simulink model "PWM_single_fixed"  (R2023a)
settings: Solver=VariableStepAuto  StartTime=0.0  StopTime=5  RelTol=1e-3
libraries: simulink x4
settings Model: Creator=Dell  LastModifiedBy=dhana
settings RTWCC: GPUComputeCapability=5.0

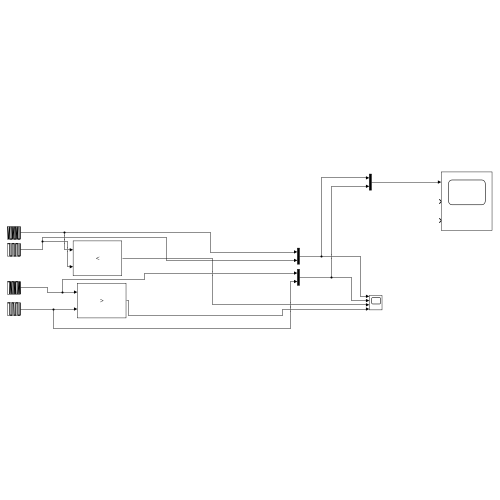
[thumbnail: Simulink's stored preview of the top-level diagram]
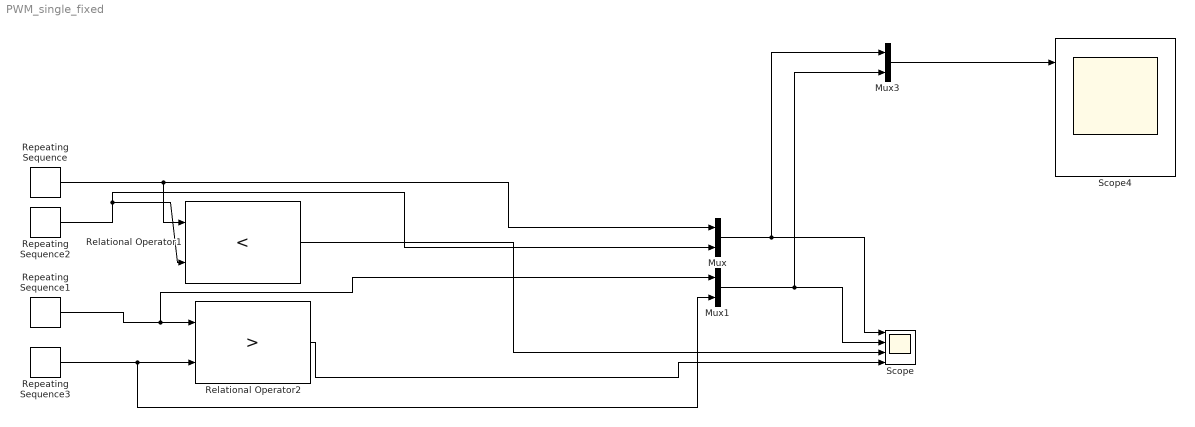
== system PWM_single_fixed ==
  Mux : Mux  Inputs=2
  Mux1 : Mux  Inputs=2
  Mux3 : Mux  Inputs=2
  Relational Operator1 : RelationalOperator  Operator=<  OutDataTypeStr=boolean  RndMeth=Simplest  InputSameDT=off
  Relational Operator2 : RelationalOperator  Operator=>  OutDataTypeStr=boolean  RndMeth=Simplest  InputSameDT=off
  Repeating Sequence : simulink/Sources/Repeating Sequence  rep_seq_t=[0 1 2 2.0001 3 4 ]  rep_seq_y=[1 0 1 0 0 0]
  Repeating Sequence1 : simulink/Sources/Repeating Sequence  rep_seq_t="[0 1 2 2.0001 3 4 4.0001  ]"  rep_seq_y=[0 0 0 -1 0 -1 0 ]
  Repeating Sequence2 : simulink/Sources/Repeating Sequence  rep_seq_t=[0 1 2 2.0001 3 4 ]  rep_seq_y=[0.8 0.8 0.8 0 0 0]
  Repeating Sequence3 : simulink/Sources/Repeating Sequence  rep_seq_t="[0 1 2 2.0001 3 4 4.0001  ]"  rep_seq_y=[0 0 0 -0.8 -0.8 -0.8 0 ]
  Scope : Scope  NumInputPorts=4
  Scope4 : Scope  NumInputPorts=3
  wires:
  Repeating Sequence/1 -> Mux/1, Relational Operator1/1
  Repeating Sequence2/1 -> Mux/2, Relational Operator1/2
  Repeating Sequence3/1 -> Mux1/2, Relational Operator2/2
  Repeating Sequence1/1 -> Mux1/1, Relational Operator2/1
  Mux3/1 -> Scope4/1
  Mux1/1 -> Mux3/2, Scope/2
  Mux/1 -> Mux3/1, Scope/1
  Relational Operator1/1 -> Scope/3
  Relational Operator2/1 -> Scope/4
